simulink model "mpc_based_model"  (R2021a)
settings: Solver=VariableStepAuto  StartTime=0.0  StopTime=240  RelTol=1e-3
undefined symbols (not defined in the file or in its folder): sigbuilder_block
libraries: mpcadaslib x1
settings Model: Creator=uddin  LastModifiedBy=uddin

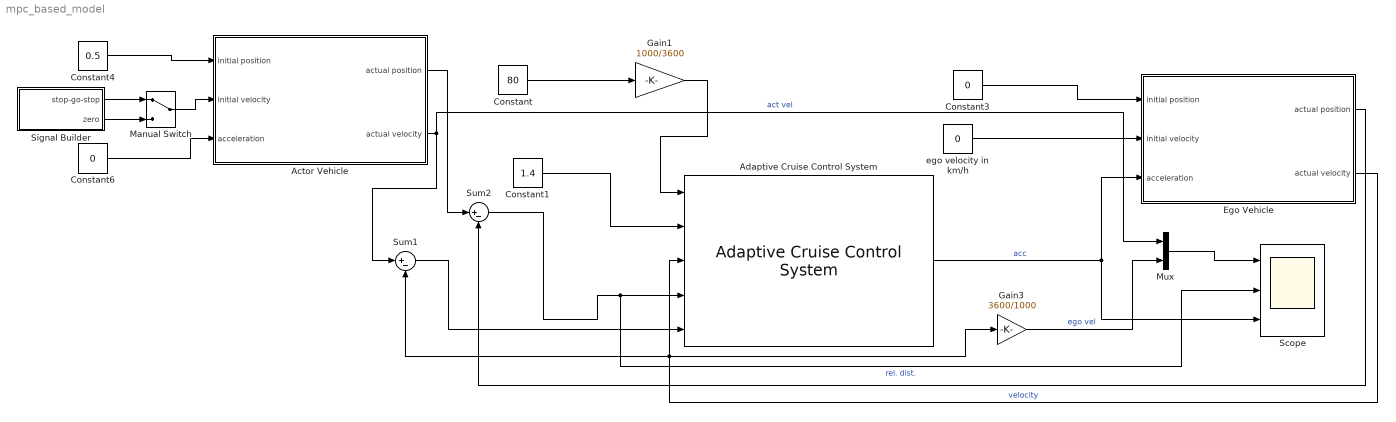
== system mpc_based_model ==
  Actor Vehicle : Subsystem
  Adaptive Cruise Control System : mpcadaslib/Adaptive Cruise Control System  EgoModel=tf(1,[0.5,1,0])  InitialEgoVelocity=0  DefaultSpacing=0.5  MaxVelocity=120*1000/3600  MinAcceleration=-3  amin_ext=off  MaxAcceleration=2  amax_ext=off  Ts=1  PredictionHorizon=15  ControllerBehavior=0.0  suboptimal=off  maxiter=20  datatypeopt=double  optmode=off  trackmode=off
  Constant : Constant  Value=80  SampleTime=1
  Constant1 : Constant  Value=1.4  SampleTime=1
  Constant3 : Constant  Value=0  SampleTime=1
  Constant4 : Constant  Value=0.5  SampleTime=1
  Constant6 : Constant  Value=0  SampleTime=1
  Ego Vehicle : Subsystem
  Gain1 : Gain  Gain=1000/3600
  Gain3 : Gain  Gain=3600/1000
  Manual Switch : ManualSwitch
  Mux : Mux  Inputs=2
  Scope : Scope  NumInputPorts=3
  Signal Builder : Subsystem  Tag=STV Subsys  LoadFcn=sigbuilder_block('load');  StartFcn=sigbuilder_block('start');  StopFcn=sigbuilder_block('stop');  ClipboardFcn=sigbuilder_block('clipboard');  mask(Sigbuilder block){tuvar=[0:10]}
      mask help: Simulink:masks:SigbuilderBlock_MD
      mask init:
      | if ~strcmp(get_param(bdroot(gcbh),'SimulationStatus'),'stopped') tuvar = sigbuilder_block('maskInit'); end
      settings: CopyFcn=sigbuilder_block('copy');  DeleteFcn=sigbuilder_block('delete');  ModelCloseFcn=sigbuilder_block('modelClose');  PreSaveFcn=sigbuilder_block('preSave');  PauseFcn=sigbuilder_block('pause');  ContinueFcn=sigbuilder_block('continue');  NameChangeFcn=sigbuilder_block('namechange');  OpenFcn=sigbuilder_block('open',[393 134.4 550.8 400.2 ]);  CloseFcn=sigbuilder_block('close');
      mask Display: plot(0, 0, 100, 100,[2, 2, 32, 32, 2], [68, 8, 8, 68, 68],[32, 2], [38, 38], [32, 19, 2],[53, 60, 44], [32, 17, 17, 2],[16, 16, 31, 31]);txt = getActiveGroup(gcbh);text(2, 100, txt,'verticalAlignment', 'top');
  Sum1 : Sum  Inputs=|+-
  Sum2 : Sum  Inputs=|+-
  ego velocity in km/h : Constant  Value=0  SampleTime=1
  wires:
  Constant1/1 -> Adaptive Cruise Control System/2
  Sum2/1 -> Adaptive Cruise Control System/4, Scope/2  "rel. dist."
  Sum1/1 -> Adaptive Cruise Control System/5
  Constant3/1 -> Ego Vehicle/1(initial position)
  Adaptive Cruise Control System/1 -> Scope/3, Ego Vehicle/3(acceleration)  "acc"
  Ego Vehicle/1(actual position) -> Sum2/2
  Ego Vehicle/2(actual velocity) -> Gain3/1, Adaptive Cruise Control System/3, Sum1/2  "velocity"
  Constant4/1 -> Actor Vehicle/1(initial position)
  Actor Vehicle/1(actual position) -> Sum2/1
  Constant6/1 -> Actor Vehicle/3(acceleration)
  ego velocity in km/h/1 -> Ego Vehicle/2(initial velocity)
  Constant/1 -> Gain1/1
  Gain1/1 -> Adaptive Cruise Control System/1
  Actor Vehicle/2(actual velocity) -> Sum1/1, Mux/1  "act vel"
  Gain3/1 -> Mux/2  "ego vel"
  Mux/1 -> Scope/1
  Signal Builder/1(stop-go-stop) -> Manual Switch/1
  Signal Builder/2(zero) -> Manual Switch/2
  Manual Switch/1 -> Actor Vehicle/2(initial velocity)

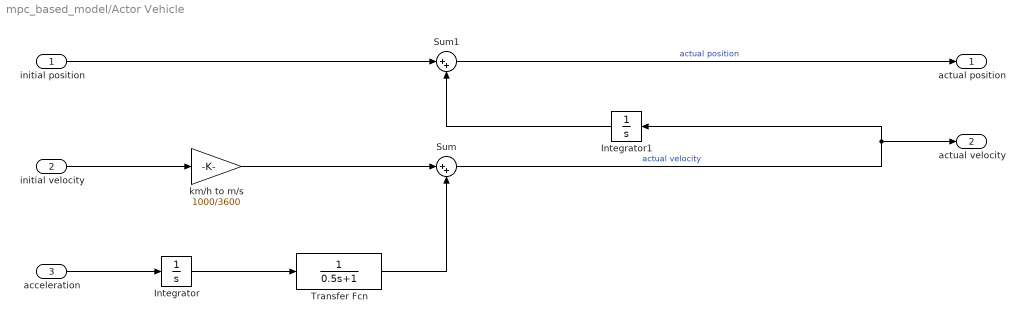
== system mpc_based_model/Actor Vehicle ==
  initial position : Inport
  initial velocity : Inport  Port=2
  acceleration : Inport  Port=3
  Integrator : Integrator  ZeroCross=off
  Integrator1 : Integrator  ZeroCross=off
  Sum : Sum  Inputs=|++
  Sum1 : Sum  Inputs=|++
  Transfer Fcn : TransferFcn  Denominator=[0.5 1]
  km/h to m/s : Gain  Gain=1000/3600
  actual position : Outport
  actual velocity : Outport  Port=2
  wires:
  Integrator1/1 -> Sum1/2
  initial position/1 -> Sum1/1
  acceleration/1 -> Integrator/1
  Sum/1 -> Integrator1/1, actual velocity/1  "actual velocity"
  Sum1/1 -> actual position/1  "actual position"
  Integrator/1 -> Transfer Fcn/1
  Transfer Fcn/1 -> Sum/2
  initial velocity/1 -> km/h to m/s/1
  km/h to m/s/1 -> Sum/1

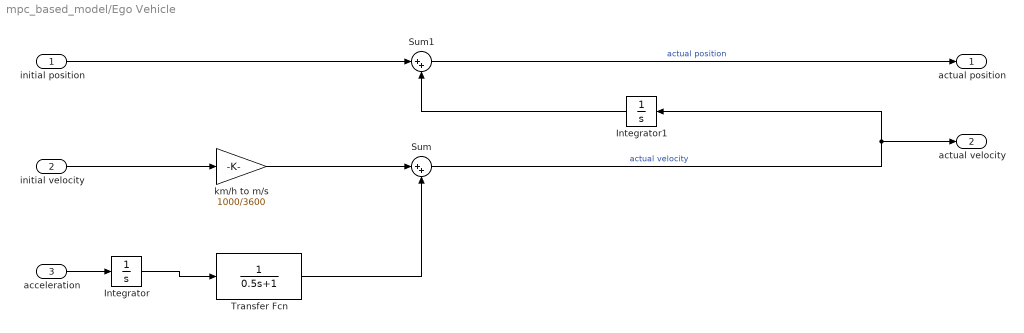
== system mpc_based_model/Ego Vehicle ==
  initial position : Inport
  initial velocity : Inport  Port=2
  acceleration : Inport  Port=3
  Integrator : Integrator  ZeroCross=off
  Integrator1 : Integrator  ZeroCross=off
  Sum : Sum  Inputs=|++
  Sum1 : Sum  Inputs=|++
  Transfer Fcn : TransferFcn  Denominator=[0.5 1]
  km/h to m/s : Gain  Gain=1000/3600
  actual position : Outport
  actual velocity : Outport  Port=2
  wires:
  Sum1/1 -> actual position/1  "actual position"
  Sum/1 -> actual velocity/1, Integrator1/1  "actual velocity"
  acceleration/1 -> Integrator/1
  initial position/1 -> Sum1/1
  Integrator1/1 -> Sum1/2
  Integrator/1 -> Transfer Fcn/1
  Transfer Fcn/1 -> Sum/2
  initial velocity/1 -> km/h to m/s/1
  km/h to m/s/1 -> Sum/1

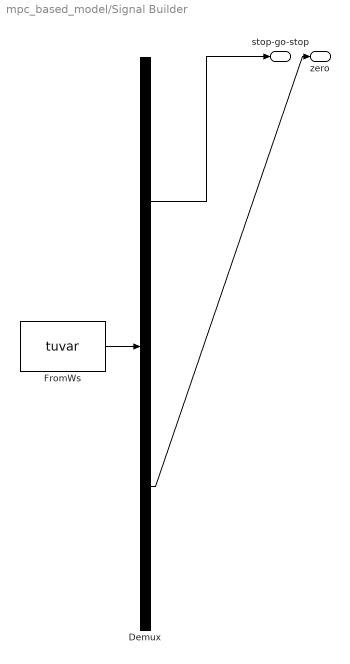
== system mpc_based_model/Signal Builder ==
  Demux : Demux  Tag=STV Demux  Outputs=2
      settings: DisplayOption=none
  FromWs : FromWorkspace  Tag=STV FromWs  VariableName=tuvar
      SigBuilderData=|
      | common.afterFinalStr = 'Extrapolate'
      | common.sampleTime = 0
      | dataSet.timeRange = [0 30]
      | dataSet.name = 'Group 1'
      | sbobj.Groups.Name = 'Group 1'
      | sbobj.Groups.Signals(1).Name = 'stop-go-stop'
      | sbobj.Groups.Signals(1).XData = [0 5 10 20 25 30]
      | sbobj.Groups.Signals(1).YData = [0 0 2 2 0 0]
      | sbobj.Groups.Signals(2).Name = 'zero'
      | sbobj.Groups.Signals(2).XData = [0 30]
      | sbobj.Groups.Signals(2).YData = [0 0]
      | sbobj.Groups.TimeRange = [0 30]
  stop-go-stop : Outport  Tag=STV Outport
  zero : Outport  Tag=STV Outport  Port=2
  wires:
  FromWs/1 -> Demux/1
  Demux/1 -> stop-go-stop/1
  Demux/2 -> zero/1
